simulink model "Copy_of_PID_2"  (R2017a)
settings: Solver=ode5  StartTime=0.0  StopTime=30  FixedStep=0.05  MaxStep=0.05  RelTol=1e-3
libraries: simulink x1
settings Model: Creator=asus  LastModifiedBy=Lenovo

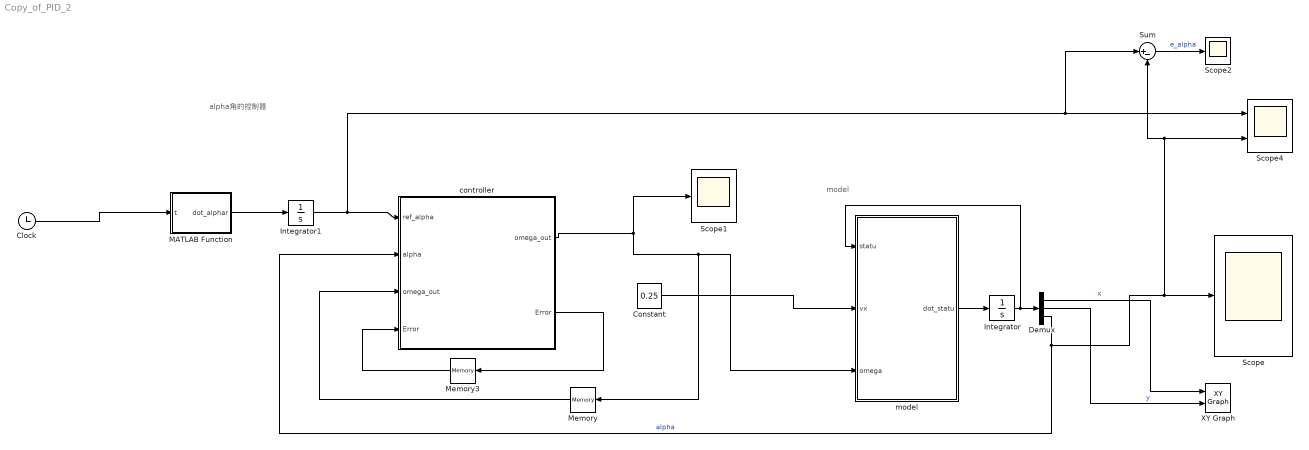
== system Copy_of_PID_2 ==
  note: alpha角的控制器
  note: model
  Clock : Clock
  Constant : Constant  Value=0.25
  Demux : Demux  Outputs=3
  Integrator : Integrator  InitialCondition=[0 0 -pi/2]  IgnoreLimit=on
  Integrator1 : Integrator  InitialCondition=pi/2
  MATLAB Function : MATLAB Function  TreatAsAtomicUnit=on
  Memory : Memory
  Memory3 : Memory  X0=[0 0]
  Scope : Scope
  Scope1 : Scope
  Scope2 : Scope
  Scope4 : Scope  NumInputPorts=2
  Sum : Sum  Inputs=|+-
  XY Graph : simulink/Sinks/XY Graph  xmin=-5  xmax=5  ymin=-5  ymax=5  st=-1
  controller : MATLAB Function  TreatAsAtomicUnit=on
  model : MATLAB Function  TreatAsAtomicUnit=on
  wires:
  Integrator/1 -> model/1(statu), Demux/1
  model/1(dot_statu) -> Integrator/1
  controller/1(omega_out) -> model/3(omega), Memory/1, Scope1/1
  Memory/1 -> controller/3("omega_out ")
  controller/2(Error) -> Memory3/1
  Memory3/1 -> controller/4("Error ")
  MATLAB Function/1(dot_alphar) -> Integrator1/1
  Sum/1 -> Scope2/1  "e_alpha"
  Integrator1/1 -> Sum/1, Scope4/1, controller/1(ref_alpha)
  Constant/1 -> model/2(vx)
  Demux/3 -> Scope4/2, Sum/2, Scope/1, controller/2(alpha)  "alpha"
  Demux/2 -> XY Graph/2  "y"
  Demux/1 -> XY Graph/1  "x"
  Clock/1 -> MATLAB Function/1(t)

== matlab function Copy_of_PID_2/controller ==
  data: ref_alpha input; omega_out output; alpha input; omega_out input; Error input; Error output
function [omega_out,Error] = my_alpha_controller( ref_alpha, alpha, omega_out,Error)
% 程序上没有问题，在运动学模型上是可以完成任务的
% 最近修改时间：11. 20
% 基于运动学模型的   控制器
% u_out=[vx ;  omega]
% ref_vel=[xr yr alphar vr omegar]
% % e = [ex ey ealpha]
% 
% 

%% 状态量                                                                           
alpha = alpha;   alphar=ref_alpha;

e2k=alphar-alpha;

e2k_1=Error(1);
e2k_2=Error(2);


kp2=15;  ki2=10;  kd2=10;
delta_u2=kp2*(e2k-e2k_1)+ki2*e2k+kd2*(e2k-2*e2k_1+e2k_2);

omega_out=delta_u2+omega_out;

e2k_2=e2k_1;
e2k_1=e2k;

Error=[e2k_1;e2k_2];
end



































% %% 测试是否能得到
% %    statu=[2; -2; pi/2; 0.001; 0.001; 0.001];
% %    u_out=[0; 0];
% %    ref_pos=[0;0;pi/4]; ref_vel=[2; 0; 0];  
% %    Error=[0 0 0 0];
% %% 底盘参数
% % d = 0.18;	l = 0.16;	m = 24;	Iz = 11.89;	c = 513.6; %轮胎侧偏刚度
% 
% %% 状态量                                                                           
% x = statu(1);   y = statu(2);  alpha = statu(3); 
% vx = statu(4);  vy = statu(5);    omega = statu(6);
% 
% xr=ref_pos(1);  yr=ref_pos(2);  alphar=ref_pos(3);
% vxr=ref_vel(1); vyr=ref_vel(2); omegar=ref_vel(3);
% 
% % e1k_1=Error(1); e1k_2=Error(2);
% 
% e2k_1=Error(3); e2k_2=Error(4);
%                                                                                       
% %%  误差
% ex=x-xr;    ey=y-yr;    ealpha=alpha-alphar;
% ev=vx-vxr;  eomega=omega-omegar;
% 
% e1k=ex+ey;
% % kp1=  0.4  ;   ki1= 0.4   ;   kd1=  0.4  ;
% % delta_u1=kp1*(e1k-e1k_1)+ki1*e1k+kd1*(e1k-2*e1k_1+e1k_2);
% 
% e2k=ealpha;
% kp2=0.4;  ki2=0.4;  kd2=0.4;
% delta_u2=kp2*(e2k-e2k_1)+ki2*e2k+kd2*(e2k-2*e2k_1+e2k_2);
% 
% delta_uout=[delta_u1;delta_u2];
% 
% u_out = delta_uout+u_out;
% 
% e1k_2=e1k_1;
% e1k_1=e1k;
% 
% e2k_2=e2k_1;
% e2k_1=e2k;
% 
% Error=[e1k_1;   e1k_2;   e2k_1 ;   e2k_2];
% 
% 
%

== matlab function Copy_of_PID_2/model ==
  data: statu input; vx input; dot_statu output; omega input
function dot_statu  = model(statu,vx,omega)

x = statu(1);
y = statu(2);
alpha = statu(3);


dot_alpha = omega;
dot_x = vx*cos(alpha);
dot_y = vx*sin(alpha);


% 状态【x y alpha vx vy omega】
dot_statu = [dot_x,dot_y,dot_alpha];

end

% max=1/wheel_radius;
% for i=1:size(wheel_omega,2)
%     if wheel_omega(i)>max
%         wheel_omega(i) = max;
%     else
%         if wheel_omega(i)<-max
%             wheel_omega(i) = -max;
%         else
%             wheel_omega(i) = wheel_omega(i);
%         end
%     end
% end

== matlab function Copy_of_PID_2/MATLAB Function ==
  data: dot_alphar output; t input
function dot_alphar = fcn(t)
% alphar=pi/2;

omegar=sin(2*t);
dot_alphar=omegar;

end
